simulink model "UAV_sync_unknown"  (R2018a)
settings: Solver=ode23tb  StartTime=0.0  StopTime=40
values from neighbouring files (symbols this model uses):
  Bm = [zeros(6); eye(6)]    [UAV_sync_unknown.m]    (also in UAV_sync_unknown_Node1.m = [zeros(6,6);ones(6,6)]; UAV_sync_unknown_Node2.m)
  C_rho = 1.225    [SC42120_UAV_Preconditions.m]
  D0 = [M0 0 0 0 0 0 ... (first row only)    [SC42120_UAV_Preconditions.m]
  Derivative_gain_phi = 50    [SC42120_UAV_Preconditions.m]
  Derivative_gain_psi = 50    [SC42120_UAV_Preconditions.m]
  Derivative_gain_theta = 50    [SC42120_UAV_Preconditions.m]
  Derivative_gain_x = 50    [SC42120_UAV_Preconditions.m]
  Derivative_gain_y = 50    [SC42120_UAV_Preconditions.m]
  Derivative_gain_z = 50    [SC42120_UAV_Preconditions.m]
  G = 9.80665    [SC42120_UAV_Preconditions.m]
  g0 = [0;0;-M0*G;0;0;0]    [SC42120_UAV_Preconditions.m]
  I0 = [0.02 0 -0.01 ... (first row only)    [SC42120_UAV_Preconditions.m]
  InitWind = [0;0;0]    [SC42120_UAV_Preconditions.m]
  Kp = diag(P)    [SC42120_UAV_Preconditions.m]
  Kv = diag(V)    [SC42120_UAV_Preconditions.m]
  M0 = 10    [SC42120_UAV_Preconditions.m]
  Pm = lyap(Am',-100*eye(12))    [UAV_sync_unknown_Node1.m]    (also in UAV_sync_unknown_Node2.m = lyap(Am',100*eye(12)))
  Proportional_phi = 50    [SC42120_UAV_Preconditions.m]
  Proportional_psi = 50    [SC42120_UAV_Preconditions.m]
  Proportional_theta = 50    [SC42120_UAV_Preconditions.m]
  Proportional_x = 50    [SC42120_UAV_Preconditions.m]
  Proportional_y = 50    [SC42120_UAV_Preconditions.m]
  Proportional_z = 50    [SC42120_UAV_Preconditions.m]
  S1 = eye(6)*1    [UAV_sync_unknown.m]    (also in UAV_sync_unknown_Node1.m = eye(6))
  S2 = eye(6)*1    [UAV_sync_unknown.m]    (also in UAV_sync_unknown_Node2.m)
undefined symbols (not defined in the file or in its folder): Aero, APlane, Bxl, C, Ctr, deg, DiscIntNeverNeededParam, F, Guid, Init, Light, MIL, Path, rad, s, Trim, Utility
libraries: aerolibconvert2 x37, simulink x15, dspsigops x7, shared6dof x6, aerolibasang x4, simulink_extras x3, aerolibadyn x1, aerolibtransform2 x1, aerolibwind2 x1
(part 2 of 6)

== system UAV_sync_unknown/Node 0/VF Approach/GROUND HIT ==
  PlantData : Inport
  Bus Selector1 : BusSelector  OutputSignals=xyh
  Bus Selector3 : BusSelector  OutputSignals=PlantData
  Constant : Constant  Value=0
  Relational Operator : RelationalOperator  Operator=<=  OutDataTypeStr=boolean  RndMeth=Simplest
  Selector : Selector  InputPortWidth=3  IndexOptions=Index vector (dialog)  Indices=3  OutputSizes=1
  Stop Simulation : Stop
  wires:
  PlantData/1 -> Bus Selector3/1
  Selector/1 -> Relational Operator/1
  Bus Selector1/1 -> Selector/1  "<xyh>"
  Constant/1 -> Relational Operator/2
  Relational Operator/1 -> Stop Simulation/1
  Bus Selector3/1 -> Bus Selector1/1  "<PlantData>"

== system UAV_sync_unknown/Node 0/VF Approach/MANUAL INPUTS ==
  note: Manual control
      |
      | The switches below enable (up position) or disable (down position) the manual control in the Visual Interface sub-block.
      | (default: down)
  note: Open-loop inputs
      |
      | The switches below enables a custom input from the Workspace (timeseries data type) to the control surfaces.
  note: Trim condition
      |
      | The sub-block below allows to try the actuators configuration for a trimmed flight.
  CtrBus : Inport
  EnvData : Inport  Port=2
  VF : Inport  Port=3
  GuidData : Inport  Port=4
  Bus Creator : BusCreator  Inputs=7
  Bus Selector : BusSelector  OutputSignals=throttle,ailerons,elevator,rudder
  Bus Selector1 : BusSelector  OutputSignals=Out_references,Target_height,Target_airspeed
  "CtrBus " : InportShadow
  From Workspace1 : FromWorkspace  Commented=on  VariableName=LogData.RCIN.ElevDem_IN  SampleTime=0.001
  From Workspace2 : FromWorkspace  Commented=on  VariableName=LogData.RCIN.RuddDem_IN  SampleTime=0.001
  From Workspace3 : FromWorkspace  Commented=on  VariableName=LogData.RCIN.ThrottleDem_IN  SampleTime=0.001
  From Workspace4 : FromWorkspace  Commented=on  VariableName=LogData.RCIN.AilDem_IN  SampleTime=0.001
  Goto4 : Goto  Commented=on  GotoTag=throttle
  Manual Switch{,1..7} (8 alike) : ManualSwitch  CurrentSetting=0
  Manual_cmd{,4..6} (4 alike) : Constant  Value=0
  Trim conditions : Subsystem
  CtrBus. : Outport
  EnvData. : Outport  Port=2
  GuidData. : Outport  Port=3
  VF. : Outport  Port=4
  wires:
  Manual Switch4/1 -> Goto4/1, Bus Creator/1  "throttle"
  Manual Switch7/1 -> Bus Creator/3  "elevator"
  Manual_cmd/1 -> Manual Switch/1
  Manual_cmd4/1 -> Manual Switch1/1
  Manual Switch5/1 -> Bus Creator/2  "ailerons"
  Manual Switch6/1 -> Bus Creator/4  "rudder"
  Manual_cmd6/1 -> Manual Switch3/1
  Manual_cmd5/1 -> Manual Switch2/1
  Bus Creator/1 -> CtrBus./1
  Manual Switch1/1 -> Manual Switch5/2  "ailerons"
  Manual Switch2/1 -> Manual Switch7/2  "elevator"
  Manual Switch3/1 -> Manual Switch6/2  "rudder"
  From Workspace3/1 -> Manual Switch4/1
  Manual Switch/1 -> Manual Switch4/2
  Bus Selector/1 -> Trim conditions/1(throttle)  "<throttle>"
  Trim conditions/1(throttout) -> Manual Switch/2
  Bus Selector/2 -> Trim conditions/2(ail)  "<ailerons>"
  Bus Selector/3 -> Trim conditions/3(elev)  "<elevator>"
  Bus Selector/4 -> Trim conditions/4(rudd)  "<rudder>"
  Trim conditions/4(ruddout) -> Manual Switch3/2
  Trim conditions/2(ailout) -> Manual Switch1/2
  Trim conditions/3(elevout) -> Manual Switch2/2
  EnvData/1 -> EnvData./1
  From Workspace4/1 -> Manual Switch5/1
  From Workspace1/1 -> Manual Switch7/1
  From Workspace2/1 -> Manual Switch6/1
  GuidData/1 -> GuidData./1
  VF/1 -> VF./1
  CtrBus/1 -> Bus Selector/1
  "CtrBus "/1 -> Bus Selector1/1
  Bus Selector1/1 -> Bus Creator/5  "<Out_references>"
  Bus Selector1/2 -> Bus Creator/6  "<Target_height>"
  Bus Selector1/3 -> Bus Creator/7  "<Target_airspeed>"

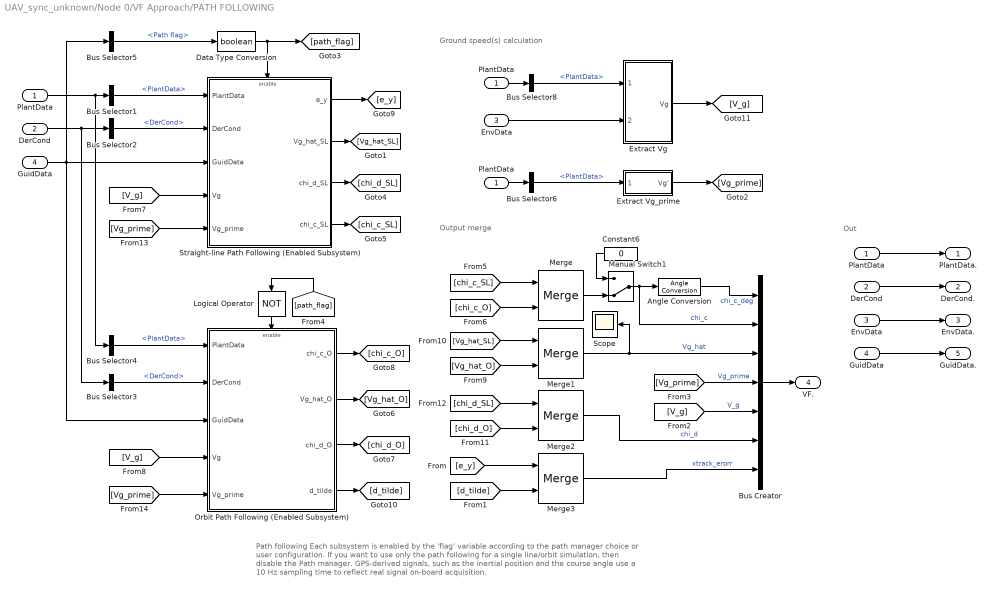
== system UAV_sync_unknown/Node 0/VF Approach/PATH FOLLOWING ==
  note: Out
  note: Ground speed(s) calculation
  note: Output merge
  note: Path following
      |
      | Each subsystem is enabled by the 'flag' variable according to the path manager choice or user configuration.
      | If you want to use only the path following for a single line/orbit simulation, then disable the Path manager.
      |
      | GPS-derived signals, such as the inertial position and the course angle use a 10 Hz sampling time to reflect real signal on-board acquisition.
  PlantData : Inport
  DerCond : Inport  Port=2
  EnvData : Inport  Port=3
  GuidData : Inport  Port=4
  Angle Conversion : aerolibconvert2/Angle Conversion  IU=rad  OU=deg
  Bus Creator : BusCreator  Inputs=7
  Bus Selector{1,4,6,8} (4 alike) : BusSelector  OutputSignals=PlantData
  Bus Selector2 : BusSelector  OutputSignals=DerCond
  Bus Selector3 : BusSelector  OutputSignals=DerCond
  Bus Selector5 : BusSelector  OutputSignals=Path flag
  Constant6 : Constant  Value=0
  Data Type Conversion : DataTypeConversion  OutDataTypeStr=boolean
  "DerCond " : InportShadow  Port=2
  "EnvData " : InportShadow  Port=3
  Extract Vg : Subsystem
  Extract Vg_prime : Subsystem
  "GuidData " : InportShadow  Port=4
  Logical Operator : Logic  Operator=NOT  AllPortsSameDT=off  OutDataTypeStr=boolean
  Manual Switch1 : ManualSwitch  CurrentSetting=0
  Merge{,1..3} (4 alike) : Merge
  Orbit Path Following (Enabled Subsystem) : Subsystem  TreatAsAtomicUnit=on
  "PlantData " : InportShadow
  "PlantData  " : InportShadow
  "PlantData   " : InportShadow
  Scope : Scope
  Straight-line Path Following (Enabled Subsystem) : Subsystem  TreatAsAtomicUnit=on
  "PlantData. " : Outport
  "DerCond. " : Outport  Port=2
  EnvData. : Outport  Port=3
  VF. : Outport  Port=4
  GuidData. : Outport  Port=5
  wires:
  Merge/1 -> Manual Switch1/2
  Constant6/1 -> Manual Switch1/1
  EnvData/1 -> EnvData./1
  PlantData/1 -> Bus Selector4/1, Bus Selector1/1
  Bus Selector1/1 -> Straight-line Path Following (Enabled Subsystem)/1(PlantData)  "<PlantData>"
  DerCond/1 -> Bus Selector2/1, Bus Selector3/1
  Bus Creator/1 -> VF./1
  Manual Switch1/1 -> Bus Creator/2, Angle Conversion/1  "chi_c"
  Logical Operator/1 -> Orbit Path Following (Enabled Subsystem)/Enable
  Bus Selector4/1 -> Orbit Path Following (Enabled Subsystem)/1(PlantData)  "<PlantData>"
  Bus Selector3/1 -> Orbit Path Following (Enabled Subsystem)/2(DerCond)  "<DerCond>"
  Data Type Conversion/1 -> [path_flag], Straight-line Path Following (Enabled Subsystem)/Enable
  [path_flag] -> Logical Operator/1
  Bus Selector2/1 -> Straight-line Path Following (Enabled Subsystem)/2(DerCond)  "<DerCond>"
  Merge1/1 -> Bus Creator/3, Scope/1  "Vg_hat"
  [Vg_prime] -> Bus Creator/4  "Vg_prime"
  Straight-line Path Following (Enabled Subsystem)/2(Vg_hat_SL) -> [Vg_hat_SL]
  Straight-line Path Following (Enabled Subsystem)/3(chi_d_SL) -> [chi_d_SL]
  Straight-line Path Following (Enabled Subsystem)/4(chi_c_SL) -> [chi_c_SL]
  Orbit Path Following (Enabled Subsystem)/2(Vg_hat_O) -> [Vg_hat_O]
  Orbit Path Following (Enabled Subsystem)/3(chi_d_O) -> [chi_d_O]
  Orbit Path Following (Enabled Subsystem)/1(chi_c_O) -> [chi_c_O]
  [chi_c_SL] -> Merge/1
  [chi_c_O] -> Merge/2
  [Vg_hat_O] -> Merge1/2
  [Vg_hat_SL] -> Merge1/1
  [chi_d_O] -> Merge2/2
  [chi_d_SL] -> Merge2/1
  Merge2/1 -> Bus Creator/6  "chi_d"
  Angle Conversion/1 -> Bus Creator/1  "chi_c_deg"
  Straight-line Path Following (Enabled Subsystem)/1(e_y) -> [e_y]
  [e_y] -> Merge3/1
  Orbit Path Following (Enabled Subsystem)/4(d_tilde) -> [d_tilde]
  [d_tilde] -> Merge3/2
  Merge3/1 -> Bus Creator/7  "xtrack_erorr"
  GuidData/1 -> Bus Selector5/1, Orbit Path Following (Enabled Subsystem)/3(GuidData), Straight-line Path Following (Enabled Subsystem)/3(GuidData)
  Bus Selector5/1 -> Data Type Conversion/1  "<Path flag>"
  "DerCond "/1 -> "DerCond. "/1
  "GuidData "/1 -> GuidData./1
  "PlantData "/1 -> "PlantData. "/1
  Extract Vg_prime/1(Vg') -> [Vg_prime]
  Bus Selector6/1 -> Extract Vg_prime/1(PlantData)  "<PlantData>"
  [V_g] -> Bus Creator/5  "V_g"
  Extract Vg/1(Vg) -> [V_g]
  "PlantData  "/1 -> Bus Selector6/1
  [V_g] -> Straight-line Path Following (Enabled Subsystem)/4(Vg)
  [V_g] -> Orbit Path Following (Enabled Subsystem)/4(Vg)
  [Vg_prime] -> Straight-line Path Following (Enabled Subsystem)/5(Vg_prime)
  [Vg_prime] -> Orbit Path Following (Enabled Subsystem)/5(Vg_prime)
  "EnvData "/1 -> Extract Vg/2(EnvData)
  "PlantData   "/1 -> Bus Selector8/1
  Bus Selector8/1 -> Extract Vg/1(PlantData)  "<PlantData>"

== system UAV_sync_unknown/Node 0/VF Approach/PATH MANAGER ==
  note: Path following only
  note: Path manager
  PlantData : Inport
  DerCond : Inport  Port=2
  EnvData : Inport  Port=3
  Bus Selector : BusSelector  OutputSignals=PlantData.Position (inertial)
  Constant : Constant  Value=Path.onOff
  Constant1 : Constant  Value=Path.onOff
  Data Type Conversion : DataTypeConversion  OutDataTypeStr=boolean
  Enabled Subsystem : Subsystem  TreatAsAtomicUnit=on
  Fcn : Fcn  Commented=on  Expr=u(1)
  Fcn1 : Fcn  Commented=on  Expr=u(2)
  Logical Operator : Logic  Operator=NOT  AllPortsSameDT=off  OutDataTypeStr=boolean
  Merge : Merge
  Path Following data : Subsystem  TreatAsAtomicUnit=on
  XY Graph : simulink/Sinks/XY Graph  Commented=on  xmin=-50  xmax=600  ymin=-50  ymax=600  st=0.1
  Plantdata. : Outport
  DerCond. : Outport  Port=2
  EnvData. : Outport  Port=3
  GuidData. : Outport  Port=4
  wires:
  PlantData/1 -> Bus Selector/1, Plantdata./1
  DerCond/1 -> DerCond./1
  EnvData/1 -> EnvData./1
  Bus Selector/1 -> Fcn1/1, Fcn/1, Enabled Subsystem/1(xy)  "<Position (inertial)>"
  Merge/1 -> GuidData./1
  Constant/1 -> Data Type Conversion/1
  Data Type Conversion/1 -> Enabled Subsystem/Enable
  Constant1/1 -> Logical Operator/1
  Logical Operator/1 -> Path Following data/Enable
  Enabled Subsystem/1(GuidData) -> Merge/1
  Path Following data/1(GuidData) -> Merge/2
  Fcn/1 -> XY Graph/1
  Fcn1/1 -> XY Graph/2

== system UAV_sync_unknown/Node 0/VF Approach/TO WORKSPACE ==
  PlantData : Inport
  DerCond : Inport  Port=2
  ControlBus : Inport  Port=3
  VF : Inport  Port=4
  GuidData : Inport  Port=5
  EnvData : Inport  Port=6
  Bus Creator : BusCreator  Inputs=6
  Bus Selector4 : BusSelector  OutputSignals=DerCond
  Bus Selector5 : BusSelector  OutputSignals=PlantData
  Sample at 0.01s : ZeroOrderHold  SampleTime=0.01
  To Workspace2 : ToWorkspace  VariableName=SimOut  SaveFormat=Timeseries  SampleTime=-1
      settings: Save2DSignal=2-D array (concatenate along first dimension)
  wires:
  Bus Creator/1 -> Sample at 0.01s/1
  Bus Selector5/1 -> Bus Creator/1  "<PlantData>"
  PlantData/1 -> Bus Selector5/1
  ControlBus/1 -> Bus Creator/3  "ControlBus"
  DerCond/1 -> Bus Selector4/1
  Bus Selector4/1 -> Bus Creator/2  "<DerCond>"
  GuidData/1 -> Bus Creator/5  "GuidData"
  VF/1 -> Bus Creator/4  "VF"
  EnvData/1 -> Bus Creator/6  "EnvData"
  Sample at 0.01s/1 -> To Workspace2/1

== system UAV_sync_unknown/Node 0/Node 0/Inverse Dynamics Control/Inverse Dynamic 1 ==
  References : Inport
  Aircraft Data : Inport  Port=2
  Add2 : Sum  Inputs=-+
  Bus Selector2 : BusSelector  OutputSignals=xyh_body,Euler angles (rad),Velocity (body),Angular rates (body)
  Bus Selector3 : BusSelector  OutputSignals=xddot_ref_final,yddot_ref_final,hddot_ref_final,phiddot_ref_final,thetaddot_ref_final,psiddot_ref_final
  Constant10 : Constant  Value=D0
  Gain3 : Gain  Gain=-1
  Inner Controller : Subsystem
  Mux1 : Mux  Inputs=6
  Mux5 : Mux  Inputs=6
  Product1 : Product  Multiplication=Matrix(*)
  Subsystem : Subsystem
  D_qddot : Outport
  wires:
  Aircraft Data/1 -> Bus Selector2/1
  Subsystem/4(e_phi) -> Inner Controller/4(e_phi)
  Subsystem/3(e_z) -> Inner Controller/3(e_z)
  Subsystem/5(e_theta) -> Inner Controller/5(e_theta)
  Bus Selector2/1 -> Subsystem/1(<xyh>)  "<xyh_body>"
  Subsystem/2(e_y) -> Inner Controller/2(e_y)
  Mux5/1 -> Add2/1
  Subsystem/6(e_psi) -> Inner Controller/6(e_psi)
  Product1/1 -> D_qddot/1
  Add2/1 -> Product1/2
  Inner Controller/3(act3) -> Gain3/1
  Constant10/1 -> Product1/1
  Mux1/1 -> Add2/2
  Bus Selector2/2 -> Subsystem/2(<Euler angles (rad)>)  "<Euler angles (rad)>"
  Inner Controller/1(act1) -> Mux5/1
  Subsystem/1(e_x) -> Inner Controller/1(e_x)
  Inner Controller/5(act5) -> Mux5/5
  Inner Controller/6(act6) -> Mux5/6
  Inner Controller/4(act4) -> Mux5/4
  Bus Selector2/3 -> Subsystem/3(velocity)  "<Velocity (body)>"
  Subsystem/7(e_xdot) -> Inner Controller/7(e_xdot)
  Bus Selector2/4 -> Subsystem/4(angular_rate)  "<Angular rates (body)>"
  Subsystem/8(e_zdot) -> Inner Controller/8(e_zdot)
  Subsystem/9(e_phidot) -> Inner Controller/9(e_phidot)
  Subsystem/10(e_thetadot) -> Inner Controller/10(e_thetadot)
  Subsystem/11(e_psidot) -> Inner Controller/11(e_psidot)
  Subsystem/12(e_ydot) -> Inner Controller/12(e_ydot)
  Inner Controller/2(act2) -> Mux5/2
  Bus Selector3/1 -> Mux1/1  "<xddot_ref_final>"
  Bus Selector3/2 -> Mux1/2  "<yddot_ref_final>"
  Bus Selector3/3 -> Mux1/3  "<hddot_ref_final>"
  Bus Selector3/4 -> Mux1/4  "<phiddot_ref_final>"
  Bus Selector3/5 -> Mux1/5  "<thetaddot_ref_final>"
  Bus Selector3/6 -> Mux1/6  "<psiddot_ref_final>"
  References/1 -> Subsystem/5(Reference), Bus Selector3/1
  Gain3/1 -> Mux5/3

== system UAV_sync_unknown/Node 0/Node 0/Inverse Dynamics Control/Inverse Dynamic 2 ==
  Aricraft Data : Inport
  Bus Selector1 : BusSelector  OutputSignals=Velocity (body),Angular rates (body)
  Constant1 : Constant  Value=I0(3)
  Constant2 : Constant  Value=I0(1)
  Constant3 : Constant  Value=M0
  Constant4 : Constant  Value=I0(5)
  Constant5 : Constant  Value=I0(9)
  Constant6 : Constant  Value=[0 0 0;0 0 0;0 0 0]
  Constant7 : Constant  Value=0
  Matrix Concatenate : Concatenate  Mode=Multidimensional array  ConcatenateDimension=2
  Matrix Concatenate1 : Concatenate  Mode=Multidimensional array  ConcatenateDimension=2
  Matrix Concatenate2 : Concatenate  Mode=Multidimensional array
  Mux1 : Mux  Inputs=2
  Product2 : Product  Multiplication=Matrix(*)
  Rot_Matrix [3x3] : Subsystem
  Trans_Matrix [3x3] : Subsystem
  p : Fcn  Expr=u(1)
  q : Fcn  Expr=u(2)
  r : Fcn  Expr=u(3)
  C_qdot : Outport
  wires:
  Aricraft Data/1 -> Bus Selector1/1
  Matrix Concatenate/1 -> Matrix Concatenate2/1
  Matrix Concatenate1/1 -> Matrix Concatenate2/2
  Rot_Matrix [3x3]/1(Out1) -> Matrix Concatenate1/2
  Constant7/1 -> Trans_Matrix [3x3]/4(zero), Rot_Matrix [3x3]/4(Zero)
  Constant3/1 -> Trans_Matrix [3x3]/5(M)
  r/1 -> Rot_Matrix [3x3]/3(r), Trans_Matrix [3x3]/3(r)
  Constant2/1 -> Rot_Matrix [3x3]/5(I1)
  Trans_Matrix [3x3]/1(Out1) -> Matrix Concatenate/1
  Bus Selector1/1 -> Mux1/1  "<Velocity (body)>"
  Constant4/1 -> Rot_Matrix [3x3]/6(I5)
  Matrix Concatenate2/1 -> Product2/1
  Bus Selector1/2 -> Mux1/2, p/1, q/1, r/1  "<Angular rates (body)>"
  Constant5/1 -> Rot_Matrix [3x3]/7(I9)
  Constant6/1 -> Matrix Concatenate/2, Matrix Concatenate1/1
  q/1 -> Rot_Matrix [3x3]/2(q), Trans_Matrix [3x3]/2(q)
  p/1 -> Rot_Matrix [3x3]/1(p), Trans_Matrix [3x3]/1(p)
  Product2/1 -> C_qdot/1
  Mux1/1 -> Product2/2
  Constant1/1 -> Rot_Matrix [3x3]/8(I3_I7)

== system UAV_sync_unknown/Node 0/VF Approach/AUTOPILOT/Fly-by-wire inputs ==
  note: Put here your custom inputs
  Thr in : Inport
  Pitch in : Inport  Port=2
  . : Inport  Port=3
  Roll in : Inport  Port=4
  Constant : Constant  Commented=on  Value=0
  Dummy port : Terminator
  From Workspace : FromWorkspace  Commented=on  VariableName=LogData.RCIN.Throttle_IN  SampleTime=0.001
  From Workspace1 : FromWorkspace  Commented=on  VariableName=LogData.RCIN.Pitch_IN  SampleTime=0.001
  From Workspace2 : FromWorkspace  Commented=on  VariableName=LogData.RCIN.Roll_IN  SampleTime=0.001
  Manual Switch1 : ManualSwitch  CurrentSetting=0
  Manual Switch2 : ManualSwitch
  Manual Switch3 : ManualSwitch
  Manual Switch4 : ManualSwitch
  Thr out : Outport
  Pitch out : Outport  Port=2
  Roll out : Outport  Port=3
  tag scope: PitchDem=scoped, RollDem=scoped, ThrottleDem=scoped
  wires:
  Manual Switch3/1 -> Pitch out/1
  Manual Switch1/1 -> Thr out/1
  Pitch in/1 -> [PitchDem], Manual Switch3/1
  From Workspace/1 -> Manual Switch1/1
  Manual Switch2/1 -> [RollDem], Roll out/1
  Roll in/1 -> Manual Switch2/1
  From Workspace1/1 -> Manual Switch3/2
  Thr in/1 -> [ThrottleDem], Manual Switch1/2
  Constant/1 -> Manual Switch4/2
  From Workspace2/1 -> Manual Switch4/1
  Manual Switch4/1 -> Manual Switch2/2
  ./1 -> Dummy port/1

== system UAV_sync_unknown/Node 0/VF Approach/AUTOPILOT/Low-level Controllers ==
  ThrottIn : Inport  Unit=%
  Pitch : Inport  Port=2  Unit=deg
  Roll : Inport  Port=3  Unit=deg
  PlantData : Inport  Port=4
  Angle Conversion1 : aerolibconvert2/Angle Conversion  IU=rad  OU=deg
  Angle Conversion2 : aerolibconvert2/Angle Conversion  IU=rad  OU=deg
  Angular Velocity Conversion : aerolibconvert2/Angular Velocity Conversion  IU=rad/s  OU=deg/s
      settings: SourceProductName=Aerospace Blockset
  Angular Velocity Conversion1 : aerolibconvert2/Angular Velocity Conversion  IU=rad/s  OU=deg/s
      settings: SourceProductName=Aerospace Blockset
  Bus Selector : BusSelector  OutputSignals=Euler angles (rad)
  Bus Selector1 : BusSelector  OutputSignals=Angular rates (body) (rad/s)
  Bus Selector2 : BusSelector  OutputSignals=Euler angles (rad)
  Bus Selector3 : BusSelector  OutputSignals=Angular rates (body) (rad/s)
  Bus Selector5 : BusSelector  OutputSignals=Angular rates (body) (rad/s)
  Bus Selector6 : BusSelector  OutputSignals=Euler angles (rad)
  Bus Selector7 : BusSelector  OutputSignals=Accelerations (body/body)
  Get scaling factor : Subsystem
  Pitch controller : Subsystem
  Roll controller : Subsystem
  Side-slip angle controller : Subsystem
  ThrottOut : Outport  Unit=%
  AilDemand : Outport  Port=2  Unit=deg
  ElevDemand : Outport  Port=3  Unit=deg
  RuddDemand : Outport  Port=4  Unit=deg
  wires:
  Bus Selector/1 -> Angle Conversion1/1  "<Euler angles (rad)>"
  Roll controller/1(AilDemand) -> [AilDem], AilDemand/1
  Bus Selector1/1 -> Angular Velocity Conversion1/1  "<Angular rates (body) (rad/s)>"
  Bus Selector2/1 -> Angle Conversion2/1  "<Euler angles (rad)>"
  Bus Selector3/1 -> Angular Velocity Conversion/1  "<Angular rates (body) (rad/s)>"
  Pitch controller/1(ElevDemand) -> ElevDemand/1
  Get scaling factor/1(Scaler) -> Roll controller/4(Scaler), Side-slip angle controller/4(Scaler), Pitch controller/4(Scaler)
  Bus Selector7/1 -> Side-slip angle controller/3(accel_y)  "<Accelerations (body/body)>"
  Bus Selector6/1 -> Side-slip angle controller/2("Euler angles ")  "<Euler angles (rad)>"
  Bus Selector5/1 -> Side-slip angle controller/1(Yaw_rate)  "<Angular rates (body) (rad/s)>"
  [PlantData] -> Bus Selector1/1, Bus Selector2/1, Bus Selector3/1, Bus Selector5/1, Bus Selector6/1, Bus Selector7/1, Bus Selector/1
  Pitch/1 -> [PitchRef]
  PlantData/1 -> [PlantData]
  ThrottIn/1 -> ThrottOut/1
  Angle Conversion2/1 -> Pitch controller/2(EulerAngles)
  Angular Velocity Conversion/1 -> Pitch controller/3(AngularRates)
  Angle Conversion1/1 -> Roll controller/2(Euler angles)
  Angular Velocity Conversion1/1 -> Roll controller/3(AngularRates)
  Roll/1 -> [RollRef]
  [PitchRef] -> Pitch controller/1(PitchReference)
  [RollRef] -> Roll controller/1(RollReference)
  [AilDem] -> Side-slip angle controller/5(AilDemand)
  Side-slip angle controller/1(RudderDemand) -> RuddDemand/1

== system UAV_sync_unknown/Node 0/VF Approach/AUTOPILOT/Navigation Controller ==
  note: Activate bias only if you have troubles with undesired settling orbits.
  ReferenceCourse : Inport  Unit=deg
  DerCond : Inport  Port=2
  Angle Conversion : aerolibconvert2/Angle Conversion  IU=rad  OU=deg
  Bias : Bias  Bias=360
  Bus Selector : BusSelector  OutputSignals=Course
  Constant : Constant  Value=45
  Discrete PID Controller : simulink/Continuous/PID Controller  Controller=PD  TimeDomain=Discrete-time  SampleTime=Ctr.TS  IntegratorMethod=Forward Euler  FilterMethod=Forward Euler  Form=Parallel  UseFilter=on  ControllerParametersSource=internal  P=Ctr.Hdg2Roll.NAV_ROLL_P  I=0.01  D=Ctr.Hdg2Roll.NAV_ROLL_D  N=2*pi*20  InitialConditionSource=internal  InitialConditionForIntegrator=0  InitialConditionForFilter=0  ExternalReset=none  LimitOutput=on  UpperSaturationLimit=45  LowerSaturationLimit=-45  LinearizeAsGain=off  AntiWindupMode=clamping  Kb=1  TrackingMode=off  Kt=1  PParamMin=[]  PParamMax=[]  IParamMin=[]  IParamMax=[]  DParamMin=[]  DParamMax=[]  NParamMin=[]  NParamMax=[]  KbParamMin=[]  KbParamMax=[]  KtParamMin=[]  KtParamMax=[]  POutMin=[]  POutMax=[]  IOutMin=[]  IOutMax=[]  DOutMin=[]  DOutMax=[]  NOutMin=[]  NOutMax=[]  KbOutMin=[]  KbOutMax=[]  KtOutMin=[]  KtOutMax=[]  IntegratorOutMin=[]  IntegratorOutMax=[]  FilterOutMin=[]  FilterOutMax=[]  SumOutMin=[]  SumOutMax=[]  SumI1OutMin=[]  SumI1OutMax=[]  SumI2OutMin=[]  SumI2OutMax=[]  SumI3OutMin=[]  SumI3OutMax=[]  SumDOutMin=[]  SumDOutMax=[]  SaturationOutMin=[]  SaturationOutMax=[]  IntegratorContinuousStateAttributes=''  IntegratorStateMustResolveToSignalObject=off  IntegratorRTWStateStorageClass=Auto  FilterContinuousStateAttributes=''  FilterStateMustResolveToSignalObject=off  FilterRTWStateStorageClass=Auto  DifferentiatorICPrevScaledInput=0  DifferentiatorOutMin=[]  DifferentiatorOutMax=[]  FilterDiffOutCoefMin=[]  FilterDiffOutCoefMax=[]  SumDenOutMin=[]  SumDenOutMax=[]  SumNumOutMin=[]  SumNumOutMax=[]  ReciprocalOutMin=[]  ReciprocalOutMax=[]  DivideOutMin=[]  DivideOutMax=[]  TunerSelectOption=Transfer Function Based (PID Tuner App)
  Manual Switch : ManualSwitch  CurrentSetting=0
  Manual Switch1 : ManualSwitch
  PID : Subsystem  Commented=on
  Scope : Scope
  Scope1 : Scope
  Scope2 : Scope  NumInputPorts=2
  Step : Step  Time=10  After=90  SampleTime=0
  Sum : Sum  Inputs=|+-
  Unwrap : Subsystem
  Unwrap1 : dspsigops/Unwrap  tol=pi  InputProcessing=Columns as channels (frame based)  running=off
  Zero-Order Hold : ZeroOrderHold  SampleTime=1/400
  BankAngle : Outport  Unit=deg
  wires:
  Bus Selector/1 -> Unwrap1/1  "<Course>"
  Discrete PID Controller/1 -> Manual Switch1/1, Scope/1
  DerCond/1 -> Bus Selector/1
  Unwrap1/1 -> Angle Conversion/1  "chi_measured"
  Sum/1 -> Scope1/1, Discrete PID Controller/1
  Angle Conversion/1 -> Sum/2, Scope2/2
  ReferenceCourse/1 -> Manual Switch/2
  Unwrap/1(Out) -> Scope2/1, Sum/1
  Manual Switch/1 -> Bias/1
  Step/1 -> Zero-Order Hold/1
  Zero-Order Hold/1 -> Manual Switch/1
  Manual Switch1/1 -> BankAngle/1
  Constant/1 -> Manual Switch1/2
  Bias/1 -> Unwrap/1(In)

== system UAV_sync_unknown/Node 0/VF Approach/AUTOPILOT/Total Energy Control System ==
  note: TECS (Total Energy Control System)
      |
      | It is meant to solve the cross-coupling between height and airspeed control. This is a simplified version of the TECS (see thesis for details). This implementation has the same theoretical behaviour of ArduPilot, but without a direct correspondence with its parameters.
  PlantData : Inport
  Target_Height : Inport  Port=2
  Target_Airspeed : Inport  Port=3
  Bus Selector1 : BusSelector  OutputSignals=xyh
  Discrete PID Controller 1 : simulink/Continuous/PID Controller  Controller=PID  TimeDomain=Discrete-time  SampleTime=Ctr.TS  IntegratorMethod=Forward Euler  FilterMethod=Forward Euler  Form=Parallel  UseFilter=on  ControllerParametersSource=internal  P=1.73635676332661  I=0.34363794334664  D=0.534286386520939  N=1.11842208231346  InitialConditionSource=internal  InitialConditionForIntegrator=0  InitialConditionForFilter=0  ExternalReset=none  LimitOutput=on  UpperSaturationLimit=100  LowerSaturationLimit=0  LinearizeAsGain=off  AntiWindupMode=clamping  Kb=1  TrackingMode=off  Kt=1  PParamMin=[]  PParamMax=[]  IParamMin=[]  IParamMax=[]  DParamMin=[]  DParamMax=[]  NParamMin=[]  NParamMax=[]  KbParamMin=[]  KbParamMax=[]  KtParamMin=[]  KtParamMax=[]  POutMin=[]  POutMax=[]  IOutMin=[]  IOutMax=[]  DOutMin=[]  DOutMax=[]  NOutMin=[]  NOutMax=[]  KbOutMin=[]  KbOutMax=[]  KtOutMin=[]  KtOutMax=[]  IntegratorOutMin=[]  IntegratorOutMax=[]  FilterOutMin=[]  FilterOutMax=[]  SumOutMin=[]  SumOutMax=[]  SumI1OutMin=[]  SumI1OutMax=[]  SumI2OutMin=[]  SumI2OutMax=[]  SumI3OutMin=[]  SumI3OutMax=[]  SumDOutMin=[]  SumDOutMax=[]  SaturationOutMin=[]  SaturationOutMax=[]  IntegratorContinuousStateAttributes=''  IntegratorStateMustResolveToSignalObject=off  IntegratorRTWStateStorageClass=Auto  FilterContinuousStateAttributes=''  FilterStateMustResolveToSignalObject=off  FilterRTWStateStorageClass=Auto  DifferentiatorICPrevScaledInput=0  DifferentiatorOutMin=[]  DifferentiatorOutMax=[]  FilterDiffOutCoefMin=[]  FilterDiffOutCoefMax=[]  SumDenOutMin=[]  SumDenOutMax=[]  SumNumOutMin=[]  SumNumOutMax=[]  ReciprocalOutMin=[]  ReciprocalOutMax=[]  DivideOutMin=[]  DivideOutMax=[]  TunerSelectOption=Transfer Function Based (PID Tuner App)
  Discrete PID Controller 2 : simulink/Continuous/PID Controller  Controller=PID  TimeDomain=Discrete-time  SampleTime=Ctr.TS  IntegratorMethod=Forward Euler  FilterMethod=Forward Euler  Form=Parallel  UseFilter=on  ControllerParametersSource=internal  P=0.0957032759552278  I=0.0036993820124705  D=0.00128202697815644  N=46.36307138661  InitialConditionSource=internal  InitialConditionForIntegrator=0  InitialConditionForFilter=0  ExternalReset=none  LimitOutput=on  UpperSaturationLimit=30  LowerSaturationLimit=-30  LinearizeAsGain=off  AntiWindupMode=clamping  Kb=1  TrackingMode=off  Kt=1  PParamMin=[]  PParamMax=[]  IParamMin=[]  IParamMax=[]  DParamMin=[]  DParamMax=[]  NParamMin=[]  NParamMax=[]  KbParamMin=[]  KbParamMax=[]  KtParamMin=[]  KtParamMax=[]  POutMin=[]  POutMax=[]  IOutMin=[]  IOutMax=[]  DOutMin=[]  DOutMax=[]  NOutMin=[]  NOutMax=[]  KbOutMin=[]  KbOutMax=[]  KtOutMin=[]  KtOutMax=[]  IntegratorOutMin=[]  IntegratorOutMax=[]  FilterOutMin=[]  FilterOutMax=[]  SumOutMin=[]  SumOutMax=[]  SumI1OutMin=[]  SumI1OutMax=[]  SumI2OutMin=[]  SumI2OutMax=[]  SumI3OutMin=[]  SumI3OutMax=[]  SumDOutMin=[]  SumDOutMax=[]  SaturationOutMin=[]  SaturationOutMax=[]  IntegratorContinuousStateAttributes=''  IntegratorStateMustResolveToSignalObject=off  IntegratorRTWStateStorageClass=Auto  FilterContinuousStateAttributes=''  FilterStateMustResolveToSignalObject=off  FilterRTWStateStorageClass=Auto  DifferentiatorICPrevScaledInput=0  DifferentiatorOutMin=[]  DifferentiatorOutMax=[]  FilterDiffOutCoefMin=[]  FilterDiffOutCoefMax=[]  SumDenOutMin=[]  SumDenOutMax=[]  SumNumOutMin=[]  SumNumOutMax=[]  ReciprocalOutMin=[]  ReciprocalOutMax=[]  DivideOutMin=[]  DivideOutMax=[]  TunerSelectOption=Transfer Function Based (PID Tuner App)
  Fcn2 : Fcn  Expr=0.5 * u(1)^2
  Fcn4 : Fcn  Expr=0.5 * u(1)^2
  Gain1 : Gain  Gain=C.g
  Gain3 : Gain  Gain=C.g
  Selector1 : Selector  InputPortWidth=3  IndexOptions=Index vector (dialog)  Indices=3  OutputSizes=1
  Sum : Sum  Inputs=|++
  Sum11 : Sum  Inputs=+-
  Sum12 : Sum  Inputs=+-
  Sum13 : Sum  Inputs=|-+
  Sum8 : Sum  Inputs=|++
  Sum9 : Sum  Inputs=|-+
  ThrottleDem : Outport
  PitchDem : Outport  Port=2
  wires:
  Discrete PID Controller 2/1 -> PitchDem/1  "pitch"
  Discrete PID Controller 1/1 -> ThrottleDem/1  "throttle"
  [Va] -> Fcn2/1
  Fcn2/1 -> Sum/2, Sum11/2  "SKE"
  PlantData/1 -> Bus Selector1/1
  Bus Selector1/1 -> Selector1/1  "<xyh>"
  Selector1/1 -> Gain1/1
  Gain1/1 -> Sum/1, Sum11/1  "SPE"
  Target_Height/1 -> Gain3/1
  Gain3/1 -> Sum12/1, Sum8/1  "SPE_c"
  Target_Airspeed/1 -> Fcn4/1
  Fcn4/1 -> Sum12/2, Sum8/2  "SKE_c"
  Sum/1 -> Sum9/1  "Specific total energy"
  Sum8/1 -> Sum9/2  "Demanded specific total energy"
  Sum9/1 -> Discrete PID Controller 1/1  "STE err"
  Sum11/1 -> Sum13/1  "Specific energy balance"
  Sum12/1 -> Sum13/2  "Demanded specific energy balance"
  Sum13/1 -> Discrete PID Controller 2/1  "SBE err"

== system UAV_sync_unknown/Node 0/VF Approach/BIXLER DYNAMICS/Actuator Dynamics ==
  In : Inport
  +-15 : Saturate  UpperLimit=15  LowerLimit=-15
  +-25 : Saturate  UpperLimit=25  LowerLimit=-25
  +-30 : Saturate  UpperLimit=30  LowerLimit=-30
  Bus Creator1 : BusCreator  Inputs='delta_ail','delta_elev','delta_rudd'
  Bus Selector : BusSelector  OutputSignals=ailerons,elevator,rudder
  Scope : Scope  NumInputPorts=2
  Transfer Fcn : TransferFcn  Numerator=[45]  Denominator=[1 45]
  Transfer Fcn1 : TransferFcn  Numerator=[45]  Denominator=[1 45]
  Transfer Fcn2 : TransferFcn  Numerator=[45]  Denominator=[1 45]
  Out : Outport  Unit=deg
  wires:
  +-30/1 -> Bus Creator1/1  "delta_ail"
  Bus Creator1/1 -> Out/1  "ControlActions"
  +-25/1 -> Bus Creator1/3  "delta_rudd"
  +-15/1 -> Bus Creator1/2  "delta_elev"
  Bus Selector/2 -> Transfer Fcn1/1  "<elevator>"
  Bus Selector/1 -> Scope/1, Transfer Fcn/1  "<ailerons>"
  Bus Selector/3 -> Transfer Fcn2/1  "<rudder>"
  In/1 -> Bus Selector/1
  Transfer Fcn/1 -> Scope/2, +-30/1
  Transfer Fcn1/1 -> +-15/1
  Transfer Fcn2/1 -> +-25/1

== system UAV_sync_unknown/Node 0/VF Approach/BIXLER DYNAMICS/Derived Conditions ==
  note: WAE = Wind Angle Error
  EnvData : Inport
  PlantData : Inport  Port=2
  Angle Conversion : aerolibconvert2/Angle Conversion  IU=rad  OU=deg
  Bus Selector : BusSelector  OutputSignals=Wind total (body)
  Bus Selector1 : BusSelector  OutputSignals=Velocity (body),Velocity (inertial)
  Bus Selector2 : BusSelector  OutputSignals=Euler angles (rad)
  Constant : Constant  Value=C.rho
  Dynamic Pressure : aerolibasang/Dynamic Pressure
  "Incidence, Sideslip, & Airspeed" : aerolibasang/Incidence, Sideslip, & Airspeed
      settings: SourceProductName=Aerospace Blockset
  Scope : Scope
  Selector : Selector  InputPortWidth=3  IndexOptions=Index vector (dialog)  Indices=3  OutputSizes=1
  Selector1 : Selector  InputPortWidth=3  IndexOptions=Index vector (dialog)  Indices=2  OutputSizes=1
  Selector3 : Selector  InputPortWidth=3  IndexOptions=Index vector (dialog)  Indices=1  OutputSizes=1
  Sum2 : Sum  Inputs=|-+
  Sum4 : Sum  Inputs=+-|
  Sum5 : Sum  Inputs=+-|
  Trigonometric Function1 : Trigonometry  Operator=atan2
  qbar : Outport  Unit=kg/m/s^2
  alpha : Outport  Port=2  Unit=rad
  beta : Outport  Port=3  Unit=rad
  Va : Outport  Port=4  Unit=m/s
  CourseAngle : Outport  Port=5  Unit=rad
  CrabAngle : Outport  Port=6  Unit=rad
  WAE : Outport  Port=7  Unit=rad
  wires:
  Dynamic Pressure/1 -> qbar/1
  Bus Selector1/1 -> Sum2/2, Dynamic Pressure/1  "<Velocity (body)>"
  "Incidence, Sideslip, & Airspeed"/2 -> [beta], beta/1
  "Incidence, Sideslip, & Airspeed"/3 -> Va/1
  Bus Selector/1 -> Sum2/1  "<Wind total (body)>"
  EnvData/1 -> Bus Selector/1
  Constant/1 -> Dynamic Pressure/2
  Sum2/1 -> "Incidence, Sideslip, & Airspeed"/1  "V_a_vector"
  "Incidence, Sideslip, & Airspeed"/1 -> alpha/1
  PlantData/1 -> Bus Selector2/1, Bus Selector1/1
  Bus Selector2/1 -> Selector/1  "<Euler angles (rad)>"
  Selector/1 -> Sum4/2  "psi"
  Selector1/1 -> Trigonometric Function1/1  "V_gy"
  Bus Selector1/2 -> Selector3/1, Selector1/1  "<Velocity (inertial)>"
  Sum4/1 -> Sum5/1, CrabAngle/1
  Sum5/1 -> WAE/1
  [beta] -> Sum5/2
  Selector3/1 -> Trigonometric Function1/2  "V_gx"
  Trigonometric Function1/1 -> Sum4/1, CourseAngle/1, Angle Conversion/1
  Angle Conversion/1 -> Scope/1

== system UAV_sync_unknown/Node 0/VF Approach/BIXLER DYNAMICS/RUBBISH BIN ==
  Angle Conversion1 : aerolibconvert2/Angle Conversion  Commented=on  IU=deg  OU=rad
  Clock : Clock  Commented=on
  Constant1 : Constant  Commented=on  Value=0
  From1 : From  Commented=on  GotoTag=throttle
  From2 : From  Commented=on  GotoTag=Target_Height  TagVisibility=global
  From3 : From  Commented=on  GotoTag=Target_Airspeed  TagVisibility=global
  From7 : From  Commented=on  GotoTag=throttle
  From9 : From  Commented=on  GotoTag=PlantData
  Orbit : Subsystem  Commented=on
  Reference Signals : Subsystem  Commented=on
  Reference Signals1 : Subsystem  Commented=on
  Straight Line : Subsystem  Commented=on
  Switch : Switch  Commented=on  Criteria=u2 > Threshold  Threshold=50
  TECS : Subsystem  Commented=on
  Vector Field : MATLAB Function  Commented=on  TreatAsAtomicUnit=on
  wires:
  From7/1 -> Reference Signals/1(Throttle)
  Clock/1 -> Switch/2
  Constant1/1 -> Angle Conversion1/1
  Angle Conversion1/1 -> Switch/3
  Vector Field/1(y) -> Switch/1
  From1/1 -> Reference Signals1/1(Throttle)
  From2/1 -> TECS/3(HeightDemand)
  From3/1 -> TECS/2(TAS_dem)
  From9/1 -> TECS/1(PlantData)

== system UAV_sync_unknown/Node 0/VF Approach/BIXLER DYNAMICS/Sampling ==
  Cont. : Inport
  Bus Creator : BusCreator  Inputs=3
  Zero-Order Hold : ZeroOrderHold  SampleTime=1/400
  Zero-Order Hold1 : ZeroOrderHold  SampleTime=1/10
  Cont.+Disc. : Outport
  wires:
  Cont./1 -> Zero-Order Hold1/1, Zero-Order Hold/1, Bus Creator/3  "PlantData"
  Bus Creator/1 -> Cont.+Disc./1
  Zero-Order Hold1/1 -> Bus Creator/2  "PlantData @10Hz"
  Zero-Order Hold/1 -> Bus Creator/1  "PlantData @400Hz"

== system UAV_sync_unknown/Node 0/VF Approach/BIXLER DYNAMICS/Sampling  ==
  Cont. : Inport
  Bus Creator : BusCreator  Inputs=3
  Zero-Order Hold : ZeroOrderHold  SampleTime=1/400
  Zero-Order Hold1 : ZeroOrderHold  SampleTime=1/10
  Cont.+Disc. : Outport
  wires:
  Zero-Order Hold/1 -> Bus Creator/1  "DerCond @400Hz"
  Zero-Order Hold1/1 -> Bus Creator/2  "DerCond @10Hz"
  Bus Creator/1 -> Cont.+Disc./1
  Cont./1 -> Bus Creator/3, Zero-Order Hold/1, Zero-Order Hold1/1  "DerCond"

== system UAV_sync_unknown/Node 0/VF Approach/BIXLER DYNAMICS/Throttle Dynamics ==
  In : Inport  Unit=%
  0-100 : Saturate  UpperLimit=100  LowerLimit=0
  Transfer Fcn2 : TransferFcn  Numerator=[45]  Denominator=[1 45]
  Out : Outport  Unit=%
  wires:
  In/1 -> Transfer Fcn2/1
  0-100/1 -> Out/1
  Transfer Fcn2/1 -> 0-100/1

== system UAV_sync_unknown/Node 0/VF Approach/BIXLER DYNAMICS/Vehicle Airframe ==
  Throttle_cmd : Inport  Unit=%
  ControlActions : Inport  Port=2
  DerCond : Inport  Port=3
  6DOF (Euler Angles) : shared6dof/6DOF (Euler Angles)  units=Metric (MKS)  mtype=Fixed  rep=Euler Angles  xme_0=Init.xyz  Vm_0=Init.uvw  eul_0=deg2rad(Init.attitude)  pm_0=deg2rad(Init.pqr)  mass_0=Bxl.mass  mass_e=0.5  mass_f=2.0  inertia=Bxl.J  inertia_e=eye(3)  inertia_f=2*eye(3)  k_quat=1.0  vre_flag=on  abi_flag=off  aMode=aMode
      settings: SourceProductBaseCode=AE
  Aerodynamics : Subsystem
  Bus Creator : BusCreator  Inputs=Velocity (inertial),Position (inertial),xyh,Euler angles (rad),ome_e,Angular rates (body) (rad/s),From inertial to body matrix,Velocity (body),Angular accelerations (body/body),Accelerations (body/body),xyh_body
  "DerCond " : InportShadow  Port=3
  Gain : Gain  Gain=[1 1 -1]
  Gravity Force : Subsystem
  Product : Product  Multiplication=Matrix(*)
  Propulsion : Subsystem
  Sum : Sum
  Sum1 : Sum  Inputs=+++|
  to Omega_e : Subsystem
  PlantData : Outport
  wires:
  [DCM] -> Product/1, Bus Creator/7  "From inertial to body matrix"
  [euler] -> Bus Creator/4, to Omega_e/1(euler)  "Euler angles (rad)"
  [Vb] -> Bus Creator/8  "Velocity (body)"
  [PlantData] -> Aerodynamics/1(PlantData)
  [Ve] -> Bus Creator/1  "Velocity (inertial)"
  [Xe] -> Gain/1, Bus Creator/2  "Position (inertial)"
  [A_b] -> Bus Creator/10  "Accelerations (body/body)"
  ControlActions/1 -> Aerodynamics/3(Control)
  Sum1/1 -> 6DOF (Euler Angles)/1
  Bus Creator/1 -> PlantData/1, [PlantData]
  Sum/1 -> 6DOF (Euler Angles)/2
  [PlantData] -> Gravity Force/1(PlantData)
  Gravity Force/1(Fg) -> Sum1/1
  Throttle_cmd/1 -> Propulsion/1(Throttle)
  Propulsion/2(M) -> Sum/1
  Propulsion/1(F) -> Sum1/2
  "DerCond "/1 -> Aerodynamics/2(DerCond)
  Aerodynamics/1(AeroForces) -> Sum1/3
  Aerodynamics/2(AeroMoments) -> Sum/2
  [ome_d_b] -> Bus Creator/9  "Angular accelerations (body/body)"
  [ome_b] -> Bus Creator/6, to Omega_e/2(ome_b)  "Angular rates (body) (rad/s)"
  Gain/1 -> Product/2, Bus Creator/3  "xyh"
  to Omega_e/1(ome_e) -> Bus Creator/5  "ome_e"
  6DOF (Euler Angles)/1 -> [Ve]
  6DOF (Euler Angles)/2 -> [Xe]
  6DOF (Euler Angles)/3 -> [euler]
  6DOF (Euler Angles)/4 -> [DCM]
  6DOF (Euler Angles)/5 -> [Vb]
  6DOF (Euler Angles)/6 -> [ome_b]
  6DOF (Euler Angles)/7 -> [ome_d_b]
  6DOF (Euler Angles)/8 -> [A_b]
  DerCond/1 -> Propulsion/2(DerCond)
  Product/1 -> Bus Creator/11  "xyh_body"

== system UAV_sync_unknown/Node 0/VF Approach/ENVIRONMENT/Slowly time varying wind gen. ==
  Constant : Constant  Value=0
  Fcn : Fcn  Expr=u(1)*cos(u(2))
  Fcn1 : Fcn  Expr=u(1)*sin(u(2))
  Mux : Mux  Inputs=2
  Mux1 : Mux  Inputs=3
  Sine Wave : Sin  Amplitude=3  Frequency=0.01  SampleTime=0
  Sine Wave1 : Sin  Amplitude=pi  Frequency=0.01  SampleTime=0
  Out1 : Outport
  wires:
  Fcn/1 -> Mux1/1
  Mux1/1 -> Out1/1
  Constant/1 -> Mux1/3
  Sine Wave1/1 -> Mux/2
  Sine Wave/1 -> Mux/1
  Fcn1/1 -> Mux1/2
  Mux/1 -> Fcn1/1, Fcn/1

== system UAV_sync_unknown/Node 0/VF Approach/MANUAL INPUTS/Trim conditions ==
  note: Trim condition on/off. (default: off)
      |
      | Reminder:
      | if on, Manual Control switches must be up.
  throttle : Inport
  ail : Inport  Port=2
  elev : Inport  Port=3
  rudd : Inport  Port=4
  Manual Switch{,1..3} (4 alike) : ManualSwitch  CurrentSetting=0
  Manual_cmd1 : Constant  Value=Trim.throttle
  Manual_cmd2 : Constant  Value=Trim.ail
  Manual_cmd3 : Constant  Value=Trim.elev
  Manual_cmd7 : Constant  Value=Trim.rudd
  throttout : Outport  Unit=%
  ailout : Outport  Port=2  Unit=deg
  elevout : Outport  Port=3  Unit=deg
  ruddout : Outport  Port=4  Unit=deg
  wires:
  throttle/1 -> Manual Switch/2
  Manual_cmd1/1 -> Manual Switch/1
  Manual_cmd2/1 -> Manual Switch1/1
  Manual_cmd3/1 -> Manual Switch2/1
  Manual_cmd7/1 -> Manual Switch3/1
  ail/1 -> Manual Switch1/2
  rudd/1 -> Manual Switch3/2
  Manual Switch/1 -> throttout/1
  Manual Switch1/1 -> ailout/1
  Manual Switch2/1 -> elevout/1
  Manual Switch3/1 -> ruddout/1
  elev/1 -> Manual Switch2/2

== system UAV_sync_unknown/Node 0/VF Approach/PATH FOLLOWING/Extract Vg ==
  PlantData : Inport
  EnvData : Inport  Port=2
  10Hz : ZeroOrderHold  Commented=through  SampleTime=1/10
  "10Hz " : ZeroOrderHold  SampleTime=1/10
  Bus Selector1 : BusSelector  OutputSignals=Velocity (body)
  Bus Selector4 : BusSelector  OutputSignals=Wind velocity (dyn) (body)
  Dot Product1 : DotProduct  InputSameDT=on  OutDataTypeStr=Inherit: Inherit via internal rule
  Selector : Selector  InputPortWidth=3  IndexOptions=Index vector (dialog)  Indices=[1 2]  OutputSizes=1
  Sqrt1 : Sqrt  SaturateOnIntegerOverflow=on
  Sum2 : Sum  Inputs=|+-
  Vg : Outport
  wires:
  PlantData/1 -> Bus Selector1/1
  EnvData/1 -> 10Hz/1
  Bus Selector1/1 -> Sum2/1  "<Velocity (body)>"
  Bus Selector4/1 -> Sum2/2  "<Wind velocity (dyn) (body)>"
  Sum2/1 -> Selector/1  "Vg"
  Selector/1 -> Dot Product1/2, Dot Product1/1  "Vg_xy"
  Dot Product1/1 -> Sqrt1/1
  Sqrt1/1 -> "10Hz "/1
  "10Hz "/1 -> Vg/1
  10Hz/1 -> Bus Selector4/1

== system UAV_sync_unknown/Node 0/VF Approach/PATH FOLLOWING/Extract Vg_prime ==
  PlantData : Inport
  Bus Selector6 : BusSelector  OutputSignals=Velocity (body)
  Dot Product : DotProduct  InputSameDT=on  OutDataTypeStr=Inherit: Inherit via internal rule
  Selector : Selector  InputPortWidth=3  IndexOptions=Index vector (dialog)  Indices=[1 2]  OutputSizes=1
  Sqrt : Sqrt  SaturateOnIntegerOverflow=on
  Zero-Order Hold : ZeroOrderHold  SampleTime=1/10
  Vg' : Outport
  wires:
  Sqrt/1 -> Zero-Order Hold/1  "Vg'"
  PlantData/1 -> Bus Selector6/1
  Bus Selector6/1 -> Selector/1  "<Velocity (body)>"
  Dot Product/1 -> Sqrt/1
  Selector/1 -> Dot Product/2, Dot Product/1
  Zero-Order Hold/1 -> Vg'/1

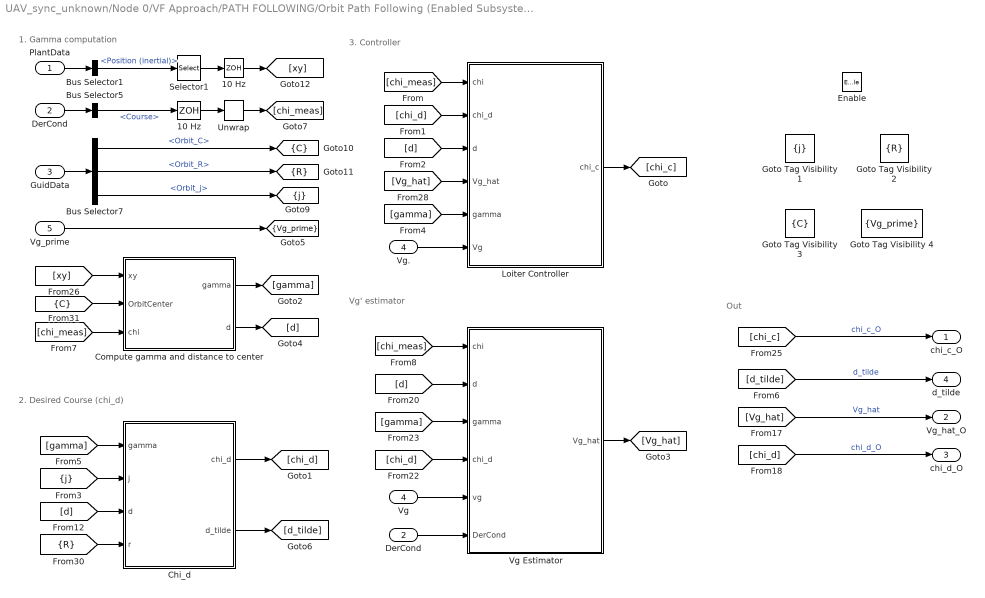
== system UAV_sync_unknown/Node 0/VF Approach/PATH FOLLOWING/Orbit Path Following (Enabled Subsystem) ==
  note: Out
  note: 3. Controller
  note: 2. Desired Course (chi_d)
  note: 1. Gamma computation
  note: Vg' estimator
  PlantData : Inport
  DerCond : Inport  Port=2
  GuidData : Inport  Port=3
  Vg : Inport  Port=4
  Vg_prime : Inport  Port=5
  Enable : EnablePort  StatesWhenEnabling=reset  PropagateVarSize=During execution
  10 Hz : ZeroOrderHold  SampleTime=1/10
  "10 Hz " : ZeroOrderHold  SampleTime=1/10
  Bus Selector1 : BusSelector  OutputSignals=Position (inertial)
  Bus Selector5 : BusSelector  OutputSignals=Course
  Bus Selector7 : BusSelector  OutputSignals=Orbit_C,Orbit_R,Orbit_j
  Chi_d : Subsystem
  Compute gamma and distance to center : Subsystem
  "DerCond " : InportShadow  Port=2
  Goto Tag Visibility 1 : GotoTagVisibility  GotoTag=j
  Goto Tag Visibility 2 : GotoTagVisibility  GotoTag=R
  Goto Tag Visibility 3 : GotoTagVisibility  GotoTag=C
  Goto Tag Visibility 4 : GotoTagVisibility  GotoTag=Vg_prime
  Loiter Controller : Subsystem
  Selector1 : Selector  InputPortWidth=3  IndexOptions=Index vector (dialog)  Indices=[1 2]  OutputSizes=1
  Unwrap : dspsigops/Unwrap  tol=pi  running=off
  Vg Estimator : Subsystem
  Vg. : InportShadow  Port=4
  chi_c_O : Outport
  Vg_hat_O : Outport  Port=2
  chi_d_O : Outport  Port=3
  d_tilde : Outport  Port=4
  tag scope: C=scoped, R=scoped, Vg_prime=scoped, j=scoped
  wires:
  Compute gamma and distance to center/1(gamma) -> [gamma]
  [Vg_hat] -> Vg_hat_O/1  "Vg_hat"
  [chi_d] -> chi_d_O/1  "chi_d_O"
  [chi_c] -> chi_c_O/1  "chi_c_O"
  Bus Selector1/1 -> Selector1/1  "<Position (inertial)>"
  Selector1/1 -> 10 Hz/1
  Compute gamma and distance to center/2(d) -> [d]
  [xy] -> Compute gamma and distance to center/1(xy)
  [gamma] -> Chi_d/1(gamma)
  [j] -> Chi_d/2(j)
  [d] -> Chi_d/3(d)
  [R] -> Chi_d/4(r)
  Chi_d/1(chi_d) -> [chi_d]
  Chi_d/2(d_tilde) -> [d_tilde]
  [chi_meas] -> Vg Estimator/1(chi)
  [d] -> Vg Estimator/2(d)
  [gamma] -> Vg Estimator/3(gamma)
  [chi_d] -> Vg Estimator/4(chi_d)
  Vg Estimator/1(Vg_hat) -> [Vg_hat]
  [chi_meas] -> Loiter Controller/1(chi)
  [chi_d] -> Loiter Controller/2(chi_d)
  [d] -> Loiter Controller/3(d)
  [Vg_hat] -> Loiter Controller/4(Vg_hat)
  [gamma] -> Loiter Controller/5(gamma)
  Loiter Controller/1(chi_c) -> [chi_c]
  DerCond/1 -> Bus Selector5/1
  "10 Hz "/1 -> Unwrap/1
  Unwrap/1 -> [chi_meas]
  [C] -> Compute gamma and distance to center/2(OrbitCenter)
  PlantData/1 -> Bus Selector1/1
  Bus Selector5/1 -> "10 Hz "/1  "<Course>"
  Vg./1 -> Loiter Controller/6(Vg)
  Vg/1 -> Vg Estimator/5(vg)
  GuidData/1 -> Bus Selector7/1
  Bus Selector7/3 -> [j]  "<Orbit_j>"
  Bus Selector7/2 -> [R]  "<Orbit_R>"
  Bus Selector7/1 -> [C]  "<Orbit_C>"
  [d_tilde] -> d_tilde/1  "d_tilde"
  Vg_prime/1 -> [Vg_prime]
  "DerCond "/1 -> Vg Estimator/6(DerCond)
  10 Hz/1 -> [xy]
  [chi_meas] -> Compute gamma and distance to center/3(chi)

== system UAV_sync_unknown/Node 0/VF Approach/PATH FOLLOWING/Straight-line Path Following (Enabled Subsystem) ==
  note: Out
  note: 3. Controller
  note: Vg' estimator
  note: 2. Desired Course (chi_d as function of e_y)
  note: 1. Crosstrack error computation
  PlantData : Inport
  DerCond : Inport  Port=2
  GuidData : Inport  Port=3
  Vg : Inport  Port=4
  Vg_prime : Inport  Port=5
  Enable : EnablePort  StatesWhenEnabling=reset  PropagateVarSize=During execution
  10 Hz : ZeroOrderHold  SampleTime=1/10
  "10 Hz " : ZeroOrderHold  SampleTime=1/10
  Bus Selector : BusSelector  OutputSignals=SL_Slope,SL_Origin
  Bus Selector1 : BusSelector  OutputSignals=Position (inertial)
  Bus Selector3 : BusSelector  OutputSignals=Course
  Chi_d : Subsystem
  Compute crosstrack error : Subsystem
  Constant1 : Constant  Value=Guid.SL.k
  Constant6 : Constant  Value=Guid.SL.chi_inf
  "DerCond " : InportShadow  Port=2
  Goto Tag Visibility : GotoTagVisibility  GotoTag=Vg_prime
  Manual Switch1 : ManualSwitch
  SL.controller : Subsystem
  Selector2 : Selector  InputPortWidth=3  IndexOptions=Index vector (dialog)  Indices=[1 2]  OutputSizes=1
  "Vg " : InportShadow  Port=4
  Vg Estimator : Subsystem
  e_y : Outport
  Vg_hat_SL : Outport  Port=2
  chi_d_SL : Outport  Port=3
  chi_c_SL : Outport  Port=4
  tag scope: Vg_prime=scoped
  wires:
  Compute crosstrack error/2(e_y) -> [e_y]
  Compute crosstrack error/1(chi_q) -> [chi_q]
  [chi_meas] -> SL.controller/1(chi)
  DerCond/1 -> Bus Selector3/1
  [chi_d] -> Manual Switch1/2
  Bus Selector/2 -> Compute crosstrack error/3(SL.Line_Origin)  "<SL_Origin>"
  [e_y] -> Chi_d/1(ey)
  [chi_q] -> Chi_d/2(chi_q)
  Constant6/1 -> Chi_d/3(chi_inf)
  Constant1/1 -> Chi_d/4(k_line)
  Chi_d/1(chi_d) -> [chi_d]
  [chi_d] -> SL.controller/2(chi_d)
  [e_y] -> SL.controller/3(e)
  [Vg_hat] -> SL.controller/4(Vg_hat)
  [chi_q] -> SL.controller/6(chi_q)
  SL.controller/1(chi_c) -> Manual Switch1/1
  GuidData/1 -> Bus Selector/1
  Bus Selector/1 -> Compute crosstrack error/2(SL.Slope)  "<SL_Slope>"
  Manual Switch1/1 -> [chi_c]  "chi_c"
  [chi_d] -> chi_d_SL/1  "chi_d_SL"
  [Vg_hat] -> Vg_hat_SL/1  "Vg_hat_SL"
  [chi_c] -> chi_c_SL/1  "chi_c_SL"
  Bus Selector3/1 -> "10 Hz "/1  "<Course>"
  PlantData/1 -> Bus Selector1/1
  Bus Selector1/1 -> Selector2/1  "<Position (inertial)>"
  Selector2/1 -> 10 Hz/1
  [xy] -> Compute crosstrack error/1(xy)
  [chi_meas] -> Vg Estimator/1(chi_meas)
  [chi_d] -> Vg Estimator/2(chi_d)
  [chi_q] -> Vg Estimator/3(chi_q)
  [e_y] -> Vg Estimator/4(e)
  Vg Estimator/1(Vg_hat) -> [Vg_hat]
  "Vg "/1 -> SL.controller/5(Vg)
  Vg/1 -> Vg Estimator/5(Vg)
  [e_y] -> e_y/1
  Vg_prime/1 -> [Vg_prime]
  "DerCond "/1 -> Vg Estimator/6(DerCond)
  10 Hz/1 -> [xy]
  "10 Hz "/1 -> [chi_meas]
  [chi_meas] -> Compute crosstrack error/4(chi)

== system UAV_sync_unknown/Node 0/VF Approach/PATH MANAGER/Enabled Subsystem ==
  xy : Inport
  Enable : EnablePort
  Bus Creator2 : BusCreator  Inputs=6
  Constant10 : Constant  Value=Path.waypoints
  Constant2 : Constant  Value=Guid.Loiter.R
  Constant3 : Constant  Value=Guid.Loiter.R
  Demux : Demux  Outputs=2
  Path Manager : MATLAB Function  TreatAsAtomicUnit=on
  Selector2 : Selector  InputPortWidth=3  IndexOptions=Index vector (dialog)  Indices=[1 2]  OutputSizes=1
  Stop Simulation : Stop
  GuidData : Outport
  wires:
  Constant10/1 -> Path Manager/1(w)
  Demux/1 -> Path Manager/2(x)
  Path Manager/6(stop_sim) -> Stop Simulation/1
  Selector2/1 -> Demux/1
  Demux/2 -> Path Manager/3(y)
  Constant2/1 -> Path Manager/4(R)
  Bus Creator2/1 -> GuidData/1
  Path Manager/1(flag) -> Bus Creator2/1  "Path flag"
  Path Manager/2(origin) -> Bus Creator2/2  "SL_Origin"
  Path Manager/3(slope) -> Bus Creator2/3  "SL_Slope"
  Path Manager/4(c) -> Bus Creator2/4  "Orbit_C"
  Constant3/1 -> Bus Creator2/5  "Orbit_R"
  Path Manager/5(lambda) -> Bus Creator2/6  "Orbit_j"
  xy/1 -> Selector2/1

== system UAV_sync_unknown/Node 0/VF Approach/PATH MANAGER/Path Following data ==
  Enable : EnablePort
  Bus Creator1 : BusCreator  Inputs=6
  Constant1 : Constant  Value=Guid.SL.Line_Origin
  Constant4 : Constant  Value=Guid.SL.Line_Slope
  Constant5 : Constant  Value=Guid.Loiter.R
  Constant6 : Constant  Value=Guid.Loiter.C
  Constant7 : Constant  Value=Guid.Loiter.j
  Constant8 : Constant  Value=Guid.Strategy
  GuidData : Outport
  wires:
  Constant1/1 -> Bus Creator1/2  "SL_Origin"
  Constant5/1 -> Bus Creator1/5  "Orbit_R"
  Constant7/1 -> Bus Creator1/6  "Orbit_j"
  Constant6/1 -> Bus Creator1/4  "Orbit_C"
  Bus Creator1/1 -> GuidData/1
  Constant8/1 -> Bus Creator1/1  "Path flag"
  Constant4/1 -> Bus Creator1/3  "SL_Slope"
